simulink model "gm_UZ_EnDat"  (R2023b)
settings: Solver=FixedStepDiscrete  StartTime=0  StopTime=0.002  RelTol=1e-3
model workspace (MAT data in the model file):
  Select = 0
libraries: hdlsllib x314, hdlmdlgenlib x10, simulink x7, simulink_extras x3
(part 1 of 7)
settings Model: SimulationMode=accelerator  PacingRate=1000  Creator=ELSYS_PC  LastModifiedBy=ELSYS_PC
settings SolverCC: AlgebraicLoopSolver=TrustRegion
settings DataIOCC: LimitDataPoints=on  SaveOutput=off  SaveTime=off
settings OptimizationCC: BlockReduction=off  ConditionallyExecuteInputs=off  DefaultParameterBehavior=Inlined  InheritOutputTypeSmallerThanSingle=on  LifeSpan=inf
settings DebuggingCC: AlgebraicLoopMsg=error  InheritedTsInSrcMsg=none  SingleTaskRateTransMsg=error  UnconnectedInputMsg=warning  UnconnectedOutputMsg=warning  UnconnectedLineMsg=warning  AllowSymbolicDim=off  StrictBusMsg=ErrorOnBusTreatedAsVector  SFUnexpectedBacktrackingDiag=warning  SFNoUnconditionalDefaultTransitionDiag=warning  SFExecutionAtInitializationDiag=none  ArithmeticOperatorsInVariantConditions=warning
settings HardwareCC: ProdBitPerPointer=32  ProdBitPerSizeT=32  ProdBitPerPtrDiffT=32  ProdLargestAtomicFloat=None  ProdIntDivRoundTo=Undefined  ProdEndianess=Unspecified  ProdWordSize=32  ProdHWDeviceType=ASIC/FPGA->ASIC/FPGA  TargetBitPerPointer=64  TargetBitPerSizeT=64  TargetBitPerPtrDiffT=64  TargetLongLongMode=on  TargetIntDivRoundTo=Zero  TargetEndianess=LittleEndian  TargetWordSize=64  TargetHWDeviceType=Custom Processor->MATLAB Host Computer  ProdEqTarget=off
settings ModelReferenceCC: EnableRefExpFcnMdlSchedulingChecks=on
settings SFSimCC: SimUseLocalCustomCode=off  CustomCodeUndefinedFunction=UseInterfaceOnly
settings RTWCC: RTWUseLocalCustomCode=off
settings CodeAppCC: StateflowObjectComments=on
settings GRTTargetCC: TargetLangStandard=C89/C90 (ANSI)  RTWCAPISignals=on  RTWCAPIParams=on
settings ConfigComp: CovScope=ReferencedModels  CovMetricSettings=dw  CovSaveCumulativeToWorkspaceVar=on  CovSaveSingleToWorkspaceVar=on  CovExternalEMLEnable=off  CovSFcnEnable=off  DVTestSuiteOptimization=Auto  DVDetectOutOfBounds=on  DVModelReferenceHarness=on  DVHarnessSource=Signal Editor  DVRebuildModelRepresentation=IfChangeIsDetected

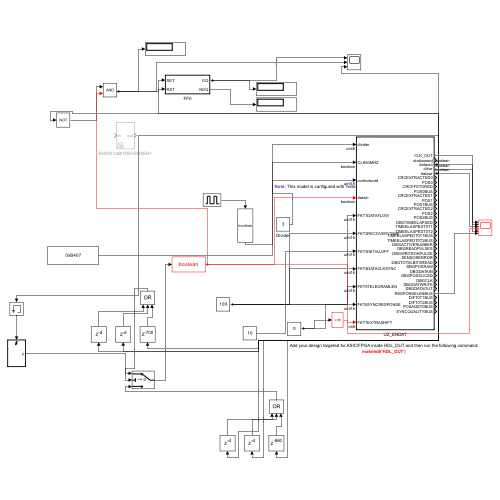
[thumbnail: Simulink's stored preview of the top-level diagram]
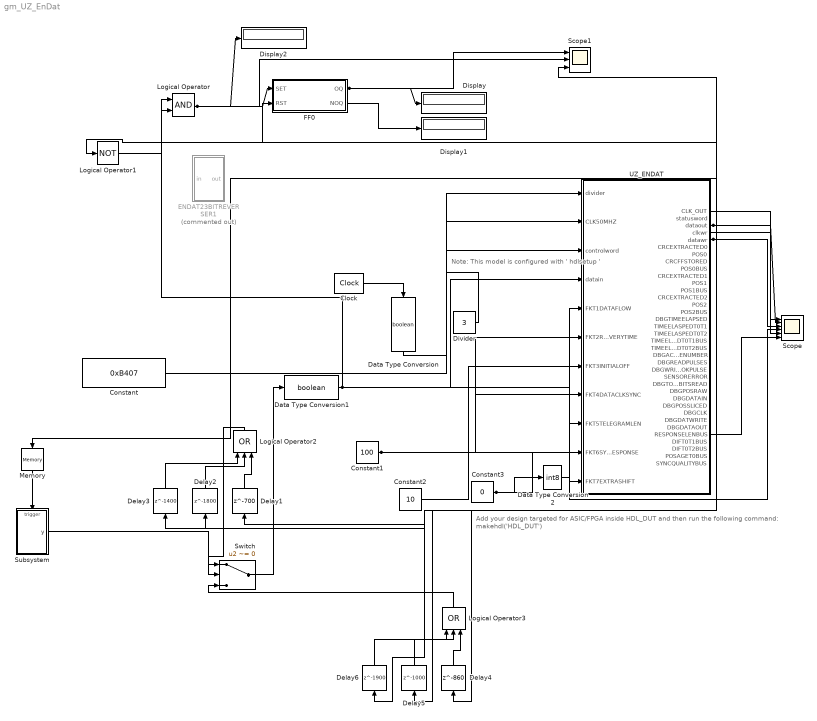
== system gm_UZ_EnDat ==
  note: Add your design targeted for ASIC/FPGA inside HDL_DUT and then run the following command:
      | makehdl('HDL_DUT')
  note: Note: This model is configured with ' hdlsetup '
  Clock : simulink_extras/Flip Flops/Clock  period=2E-8
  Constant : Constant  Value=0xB407  OutDataTypeStr=uint16  SampleTime=-1
  Constant1 : Constant  Value=100  OutDataTypeStr=uint16  SampleTime=-1
  Constant2 : Constant  Value=10  OutDataTypeStr=uint16  SampleTime=-1
  Constant3 : Constant  Value=0  OutDataTypeStr=uint16  SampleTime=-1
  Data Type Conversion : DataTypeConversion  OutDataTypeStr=boolean  SaturateOnIntegerOverflow=off  RndMeth=Floor
  Data Type Conversion1 : DataTypeConversion  OutDataTypeStr=boolean  SaturateOnIntegerOverflow=off  RndMeth=Floor
  Data Type Conversion2 : DataTypeConversion  OutDataTypeStr=int8  SaturateOnIntegerOverflow=off  RndMeth=Floor
  Delay1 : Delay  DelayLength=700
  Delay2 : Delay  DelayLength=1800
  Delay3 : Delay  DelayLength=1400
  Delay4 : Delay  DelayLength=860
  Delay5 : Delay  DelayLength=1000
  Delay6 : Delay  DelayLength=1900
  Display : Display
  Display1 : Display
  Display2 : Display
  Divider : Constant  Value=3  OutMin=0  OutMax=7  OutDataTypeStr=uint8  SampleTime=-1
  ENDAT23BITREVERSER1 : Subsystem  Commented=on
  FF0 : Subsystem  TreatAsAtomicUnit=on
      settings: LibrarySourceBlock=|
      | hdlsllib/Ports &
      | Subsystems/Triggered
      | Subsystem
  Logical Operator : Logic  AllPortsSameDT=off  OutDataTypeStr=boolean
  Logical Operator1 : Logic  Operator=NOT  AllPortsSameDT=off  OutDataTypeStr=boolean
  Logical Operator2 : Logic  Operator=OR  Inputs=3  AllPortsSameDT=off  OutDataTypeStr=boolean
  Logical Operator3 : Logic  Operator=OR  Inputs=3  AllPortsSameDT=off  OutDataTypeStr=boolean
  Memory : Memory  InheritSampleTime=on
  Scope : Scope  NumInputPorts=6
  Scope1 : Scope  NumInputPorts=3
  Subsystem : Subsystem
  Switch : Switch  Criteria=u2 ~= 0  SaturateOnIntegerOverflow=off  InputSameDT=off
  UZ_ENDAT : Subsystem  TreatAsAtomicUnit=on
  wires:
  UZ_ENDAT/32(RESPONSELENBUS) -> Scope/6
  Data Type Conversion2/1 -> UZ_ENDAT/11(FKT7EXTRASHIFT)
  Constant3/1 -> Data Type Conversion2/1, UZ_ENDAT/10(FKT6SYNCRESPONSE)
  UZ_ENDAT/4(clkwr) -> Scope/5
  Memory/1 -> Subsystem/Trigger
  Subsystem/1(y) -> Switch/2
  UZ_ENDAT/3(dataout) -> Scope/2, Delay5/1, Delay1/1, Delay2/1, Delay3/1, Delay6/1, Delay4/1
  Delay4/1 -> Logical Operator3/3
  Logical Operator3/1 -> Switch/3
  Delay5/1 -> Logical Operator3/2
  Delay6/1 -> Logical Operator3/1
  Switch/1 -> Data Type Conversion1/1
  Logical Operator2/1 -> Switch/1
  Delay3/1 -> Logical Operator2/1
  Delay2/1 -> Logical Operator2/2
  Logical Operator1/1 -> Logical Operator/1
  FF0/2(NOQ) -> Display1/1
  Logical Operator/1 -> Display2/1, FF0/1(SET), Scope1/2
  FF0/1(OQ) -> Display/1, Scope1/1
  Constant2/1 -> UZ_ENDAT/7(FKT3INITIALOFF)
  Constant1/1 -> UZ_ENDAT/9(FKT5TELEGRAMLEN), UZ_ENDAT/8(FKT4DATACLKSYNC), UZ_ENDAT/6(FKT2RECOVERYTIME), UZ_ENDAT/5(FKT1DATAFLOW)
  UZ_ENDAT/5(datawr) -> Scope/3, Logical Operator1/1, FF0/2(RST), Scope1/3, Memory/1
  UZ_ENDAT/1(CLK_OUT) -> Scope/1
  Delay1/1 -> Logical Operator2/3
  Data Type Conversion1/1 -> UZ_ENDAT/4(datain), Scope/4, Logical Operator/2
  Clock/1 -> Data Type Conversion/1
  Divider/1 -> UZ_ENDAT/1(divider)
  Data Type Conversion/1 -> UZ_ENDAT/2(CLK50MHZ)
  Constant/1 -> UZ_ENDAT/3(controlword)

== system gm_UZ_EnDat/ENDAT23BITREVERSER1 ==
  in : Inport
  16BITREVERSER : Subsystem
  16BITREVERSER1 : Subsystem
  Bit Concat : hdlsllib/Logic and Bit Operations/Bit Concat  numInputs=2
  Bit Shift : hdlsllib/Logic and Bit Operations/Bit Shift  mode=Shift Right Logical  N=8
  Bit Slice : hdlsllib/Logic and Bit Operations/Bit Slice  lidx=15  ridx=0
  Bit Slice1 : hdlsllib/Logic and Bit Operations/Bit Slice  lidx=22  ridx=16
  out : Outport
  wires:
  16BITREVERSER1/1(out) -> Bit Concat/2
  16BITREVERSER/1(out) -> Bit Concat/1
  Bit Slice1/1 -> 16BITREVERSER1/1(in)
  Bit Slice/1 -> 16BITREVERSER/1(in)
  in/1 -> Bit Slice/1, Bit Slice1/1
  Bit Shift/1 -> out/1
  Bit Concat/1 -> Bit Shift/1

== system gm_UZ_EnDat/FF0 ==
  SET : Inport
  RST : Inport  Port=2
  S-R Flip-Flop : simulink_extras/Flip Flops/S-R Flip-Flop  initial_condition=0
  OQ : Outport
  NOQ : Outport  Port=2
  wires:
  S-R Flip-Flop/2 -> NOQ/1
  S-R Flip-Flop/1 -> OQ/1
  RST/1 -> S-R Flip-Flop/2
  SET/1 -> S-R Flip-Flop/1

== system gm_UZ_EnDat/Subsystem ==
  Trigger : TriggerPort  VariantControl=(inherit)  PortDimensions=1
  Counter Limited : hdlsllib/Sources/Counter Limited  uplimit=1  tsamp=-1
  y : Outport
  wires:
  Counter Limited/1 -> y/1

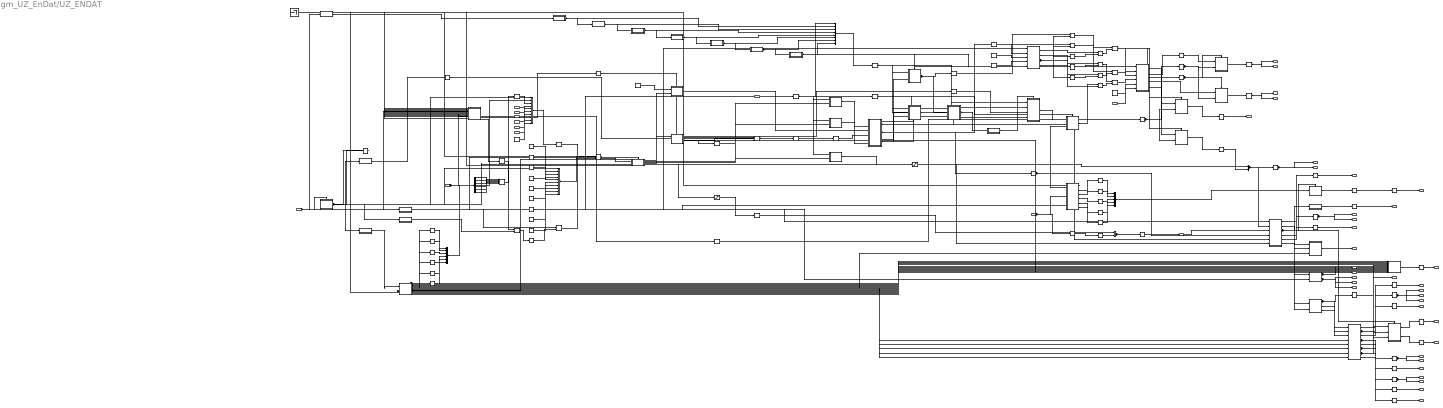
== system gm_UZ_EnDat/UZ_ENDAT ==
  note: 0=12.5;1=6,25;2=3,125;3=1,5625
  divider : Inport  OutDataTypeStr=uint8  PortDimensions=1  SampleTime=1e-08
  CLK50MHZ : Inport  Port=2  OutDataTypeStr=boolean  PortDimensions=1  SampleTime=1e-08
  controlword : Inport  Port=3  OutDataTypeStr=uint16  PortDimensions=1  SampleTime=1e-08
  datain : Inport  Port=4  OutDataTypeStr=boolean  PortDimensions=1  SampleTime=1e-08
  FKT1DATAFLOW : Inport  Port=5  OutDataTypeStr=uint16  PortDimensions=1  SampleTime=1e-08
  FKT2RECOVERYTIME : Inport  Port=6  OutDataTypeStr=uint16  PortDimensions=1  SampleTime=1e-08
  FKT3INITIALOFF : Inport  Port=7  OutDataTypeStr=uint16  PortDimensions=1  SampleTime=1e-08
  FKT4DATACLKSYNC : Inport  Port=8  OutDataTypeStr=uint16  PortDimensions=1  SampleTime=1e-08
  FKT5TELEGRAMLEN : Inport  Port=9  OutDataTypeStr=uint16  PortDimensions=1  SampleTime=1e-08
  FKT6SYNCRESPONSE : Inport  Port=10  OutDataTypeStr=uint16  PortDimensions=1  SampleTime=1e-08
  FKT7EXTRASHIFT : Inport  Port=11  OutDataTypeStr=int8  PortDimensions=1  SampleTime=1e-08
  16bitgather : Subsystem
  2CLKDELAY : simulink/Discrete/Tapped Delay  vinit=0  samptime=-1  NumDelays=double(127)  DelayOrder=Newest  includeCurrent=on
  3timestorage : Subsystem
  8BIT_SPLITTER : Subsystem
  8BIT_SPLITTER_term8 : Terminator
  CLKCNTER_ACT : Subsystem
  CLKCNTER_NOSTOP : Subsystem
  CLKDIV1 : Subsystem
  CLKDIV3 : Subsystem
  CLKDIV4 : Subsystem
  CLKDIV5 : Subsystem
  CLKDIV6 : Subsystem
  CLKDIV7 : Subsystem
  CLKDIV8 : Subsystem
  CLKDIV9 : Subsystem
  CONTROLWORDRAW : Subsystem
  CONTROLWORDRAW_term{0..11,14} (13 alike) : Terminator
  CONTROLWORDSTORED : Subsystem
  CONTROLWORDSTORED_term13 : Terminator
  CRC_Check : Subsystem
  CRC_Check_term0 : Terminator
  Compare To Constant : Subsystem  mask(Compare To Constant){relop===, const=double(1), OutDataTypeStr=boolean, ZeroCross=on}
      mask prompts: relop "Simulink:masks:Operator_MP"; const "Simulink:masks:ConstantValue_MP"; OutDataTypeStr "Simulink:masks:OutputDataType_MP"; ZeroCross "Simulink:masks:EnableZerocrossingDetection_MP"
      mask help: Simulink:masks:CompareToConstant_MD
      mask init:
      | OutDataTypeStr = 'boolean';
      | ZeroCross = 'on';
      | blkName = 'UZ_EnDat/UZ_ENDAT/Compare\nTo Constant';
      | const = double(1);
      | const_str = '1';
      | const_val = double(1);
      | relop = '==';
      | setValue = 'boolean';
      | str = '== 1';
      mask TypeOptions relop: == | ~= | < | <= | >= | >
      mask TypeOptions OutDataTypeStr: Simulink:masks:uint8 | Simulink:masks:boolean
      mask Callback ZeroCross: sl('zeroCrossEnable', gcbh);
      mask Display: disp(str)
  Compare To Constant1 : Subsystem  mask(Compare To Constant){relop===, const=double(1), OutDataTypeStr=boolean, ZeroCross=on}
      mask prompts: relop "Simulink:masks:Operator_MP"; const "Simulink:masks:ConstantValue_MP"; OutDataTypeStr "Simulink:masks:OutputDataType_MP"; ZeroCross "Simulink:masks:EnableZerocrossingDetection_MP"
      mask help: Simulink:masks:CompareToConstant_MD
      mask init:
      | OutDataTypeStr = 'boolean';
      | ZeroCross = 'on';
      | blkName = 'UZ_EnDat/UZ_ENDAT/Compare\nTo Constant1';
      | const = double(1);
      | const_str = '1';
      | const_val = double(1);
      | relop = '==';
      | setValue = 'boolean';
      | str = '== 1';
      mask TypeOptions relop: == | ~= | < | <= | >= | >
      mask TypeOptions OutDataTypeStr: Simulink:masks:uint8 | Simulink:masks:boolean
      mask Callback ZeroCross: sl('zeroCrossEnable', gcbh);
      mask Display: disp(str)
  Compare To Constant2 : Subsystem  mask(Compare To Constant){relop===, const=double(0), OutDataTypeStr=boolean, ZeroCross=on}
      mask prompts: relop "Simulink:masks:Operator_MP"; const "Simulink:masks:ConstantValue_MP"; OutDataTypeStr "Simulink:masks:OutputDataType_MP"; ZeroCross "Simulink:masks:EnableZerocrossingDetection_MP"
      mask help: Simulink:masks:CompareToConstant_MD
      mask init:
      | OutDataTypeStr = 'boolean';
      | ZeroCross = 'on';
      | blkName = 'UZ_EnDat/UZ_ENDAT/Compare\nTo Constant2';
      | const = double(0);
      | const_str = '0';
      | const_val = double(0);
      | relop = '==';
      | setValue = 'boolean';
      | str = '== 0';
      mask TypeOptions relop: == | ~= | < | <= | >= | >
      mask TypeOptions OutDataTypeStr: Simulink:masks:uint8 | Simulink:masks:boolean
      mask Callback ZeroCross: sl('zeroCrossEnable', gcbh);
      mask Display: disp(str)
  Compare To Constant3 : Subsystem  mask(Compare To Constant){relop=>=, const=double(3), OutDataTypeStr=boolean, ZeroCross=on}
      mask prompts: relop "Simulink:masks:Operator_MP"; const "Simulink:masks:ConstantValue_MP"; OutDataTypeStr "Simulink:masks:OutputDataType_MP"; ZeroCross "Simulink:masks:EnableZerocrossingDetection_MP"
      mask help: Simulink:masks:CompareToConstant_MD
      mask init:
      | OutDataTypeStr = 'boolean';
      | ZeroCross = 'on';
      | blkName = 'UZ_EnDat/UZ_ENDAT/Compare\nTo Constant3';
      | const = double(3);
      | const_str = '3';
      | const_val = double(3);
      | relop = '>=';
      | setValue = 'boolean';
      | str = '>= 3';
      mask TypeOptions relop: == | ~= | < | <= | >= | >
      mask TypeOptions OutDataTypeStr: Simulink:masks:uint8 | Simulink:masks:boolean
      mask Callback ZeroCross: sl('zeroCrossEnable', gcbh);
      mask Display: disp(str)
  Constant3 : Constant  OutDataTypeStr=boolean  SampleTime=1e-08
  Constant6 : Constant  Value=51  OutDataTypeStr=uint16  SampleTime=1e-08
  ControlWordRAM : Constant  Value=0  VectorParams1D=off  OutDataTypeStr=uint8  SampleTime=1e-08
  DATA2CLOCKSYNCER : Subsystem
  DATAFLOWCHGER : Subsystem
  DIFFBUILDER : Subsystem
  Data Type Conversion : DataTypeConversion  OutDataTypeStr=fixdt(0, 4, 0)  RndMeth=Nearest  SampleTime=1e-08
  Data Type Conversion1 : DataTypeConversion  OutDataTypeStr=uint8  SampleTime=1e-08  SaturateOnIntegerOverflow=off  RndMeth=Floor
  Data Type Conversion{2..12} (11 alike) : DataTypeConversion  OutDataTypeStr=fixdt(0, 1, 0)  SampleTime=1e-08  SaturateOnIntegerOverflow=off  RndMeth=Floor
  Delay1 : simulink/Discrete/Tapped Delay  vinit=0  samptime=-1  NumDelays=double(127)  DelayOrder=Newest  includeCurrent=on
  Delay4 : hdlmdlgenlib/Buffer
  Detect Change : Subsystem  mask(Detect Change){vinit=double(0), InputProcessing=Elements as channels (sample based), OutDataTypeStr=boolean}
      mask prompts: vinit "Simulink:masks:InitialCondition_MP"; InputProcessing "Simulink:masks:InputProcessing_MP"; OutDataTypeStr "Simulink:masks:OutputDataType_MP"
      mask help: Simulink:masks:DetectChange_MD
      mask init:
      | InputProcessing = 'Elements as channels (sample based)';
      | OutDataTypeStr = 'boolean';
      | vinit = double(0);
      mask TypeOptions InputProcessing: Simulink:masks:ColumnsAsChannelsFrameBased | Simulink:masks:ElementsAsChannelsSampleBased
      mask TypeOptions OutDataTypeStr: Simulink:masks:uint8 | Simulink:masks:boolean
      mask Display: fprintf('U ~= U/z')
  Dual Port RAM System : hdlsllib/HDL RAMs/Dual Port RAM System  RAMType=Dual port  AsyncRead=off  WriteOutputValue=New data  RAMInitialValue=0  allowBusInputs=off  WritesHaveOutput=on  NumReads=0  NumWrites=1  SimulateUsing=Code generation
  Dual Port RAM System_term0 : Terminator
  EndatControlRAM : Constant  VectorParams1D=off  OutDataTypeStr=uint8  SampleTime=1e-08
  FKT1 : Constant  Value=2  VectorParams1D=off  OutDataTypeStr=uint8  SampleTime=1e-08
  FKT2 : Constant  Value=3  VectorParams1D=off  OutDataTypeStr=uint8  SampleTime=1e-08
  FKT4 : Constant  Value=5  VectorParams1D=off  OutDataTypeStr=uint8  SampleTime=1e-08
  FKT5 : Constant  Value=6  VectorParams1D=off  OutDataTypeStr=uint8  SampleTime=1e-08
  FKT6 : Constant  Value=7  VectorParams1D=off  OutDataTypeStr=uint8  SampleTime=1e-08
  FKT7 : Constant  Value=8  VectorParams1D=off  OutDataTypeStr=uint8  SampleTime=1e-08
  INITIALOFF : Subsystem
  Logical Operator{,1,9,13..14,16,18,20} (8 alike) : Logic  AllPortsSameDT=off  OutDataTypeStr=boolean  SampleTime=1e-08
  Logical Operator{2..4,6,10,17,19,21,27} (9 alike) : Logic  Operator=NOT  Inputs=1  AllPortsSameDT=off  OutDataTypeStr=boolean  SampleTime=1e-08
  Logical Operator15 : Logic  Operator=OR  AllPortsSameDT=off  OutDataTypeStr=boolean  SampleTime=1e-08
  Logical Operator22 : Logic  Operator=OR  AllPortsSameDT=off  OutDataTypeStr=boolean  SampleTime=1e-08
  Logical Operator23 : Logic  Operator=OR  AllPortsSameDT=off  OutDataTypeStr=boolean  SampleTime=1e-08
  Logical Operator8 : Logic  Inputs=3  AllPortsSameDT=off  OutDataTypeStr=boolean  SampleTime=1e-08
  ManualSerialize : Subsystem
  Multiport Switch : MultiPortSwitch  DataPortOrder=Zero-based contiguous  Inputs=7  DiagnosticForDefault=None  zeroidx=on  SampleTime=1e-08  SaturateOnIntegerOverflow=off  InputSameDT=off
  OUTPUTCONTROLCONTINIOUS : Subsystem
  RAM_SELECTOR : MultiPortSwitch  DataPortOrder=Zero-based contiguous  Inputs=8  DataPortForDefault=Additional data port  DiagnosticForDefault=None  zeroidx=on  OutDataTypeStr=uint8  SampleTime=1e-08  SaturateOnIntegerOverflow=off  InputSameDT=off
  RAM_SELECTOR1 : MultiPortSwitch  DataPortOrder=Zero-based contiguous  Inputs=8  DataPortForDefault=Additional data port  DiagnosticForDefault=None  zeroidx=on  OutDataTypeStr=uint16  SampleTime=1e-08  SaturateOnIntegerOverflow=off  InputSameDT=off
  RECOVERYTIMESELECTOR : Subsystem
  RESPONSESLICER3X : Subsystem
  SetZeroBool : Subsystem
  SetZeroBool1 : Subsystem
  SetZeroBool2 : Subsystem
  SetZeroBool3 : Subsystem
  SetZeroBool4 : Subsystem
  SetZeroBool5 : Subsystem
  Signal Specification : SignalSpecification  OutDataTypeStr=uint16  Dimensions=1
  Storage16 : Subsystem
  Subsystem : Subsystem
  Subsystem1 : Subsystem
  Subsystem2 : Subsystem
  Subsystem6 : Subsystem
  TmpGroundAtRAM_SELECTOR1Inport10 : Constant  Value=0  VectorParams1D=off  OutDataTypeStr=uint16  SampleTime=1e-08
  TmpGroundAtRAM_SELECTORInport10 : Constant  Value=0  VectorParams1D=off  OutDataTypeStr=uint8  SampleTime=1e-08
  ageprovider : Subsystem
  concat : hdlsllib/Logic and Bit Operations/Bit Concat  numInputs=6
  concatenate : Concatenate  NumInputs=5
  concatenate1 : Concatenate  NumInputs=6
  multiportswitch : MultiPortSwitch  DataPortOrder=Zero-based contiguous  Inputs=1  DiagnosticForDefault=None  zeroidx=on  SampleTime=1e-08  SaturateOnIntegerOverflow=off  InputSameDT=off
  multiportswitch1 : MultiPortSwitch  DataPortOrder=Zero-based contiguous  Inputs=1  DiagnosticForDefault=None  zeroidx=on  SampleTime=1e-08  SaturateOnIntegerOverflow=off  InputSameDT=off
  ramselektor : Subsystem
  rd_{0,4..5,10..11,13..15,17..18} (10 alike) : Delay  DelayLength=double(1)  InitialCondition=0  SampleTime=1e-08
  rd_1 : Delay  DelayLength=double(10)  InitialCondition=0  SampleTime=1e-08
  rd_{2..3,6..9,12,16,19..25,27..31,33..35} (23 alike) : Delay  DelayLength=double(2)  InitialCondition=0  SampleTime=1e-08
  rd_26 : Delay  DelayLength=double(4)  InitialCondition=0  SampleTime=1e-08
  rd_32 : Delay  DelayLength=double(3)  InitialCondition=0  SampleTime=1e-08
  saturate : Saturate  UpperLimit=double(127)  LowerLimit=double(0)  SampleTime=1e-08  OutDataTypeStr=uint16
  saturate1 : Saturate  UpperLimit=double(127)  LowerLimit=double(0)  SampleTime=1e-08  OutDataTypeStr=uint16
  signalquality : Subsystem
  t : Constant  Value=double(0)  OutDataTypeStr=boolean  SampleTime=1e-08
  t1 : Constant  Value=fi(0,0,8,0)  OutDataTypeStr=uint8  SampleTime=1e-08
  t2 : Constant  Value=fi(0,0,16,0)  OutDataTypeStr=uint16  SampleTime=1e-08
  t3 : Demux  Outputs=6
  timingprovider : Subsystem
  CLK_OUT : Outport  SampleTime=1e-08  VectorParamsAs1DForOutWhenUnconnected=off
  statusword : Outport  Port=2  OutDataTypeStr=uint16  SampleTime=1e-08  VectorParamsAs1DForOutWhenUnconnected=off
  dataout : Outport  Port=3  OutDataTypeStr=boolean  SampleTime=1e-08  VectorParamsAs1DForOutWhenUnconnected=off
  clkwr : Outport  Port=4  OutDataTypeStr=boolean  SampleTime=1e-08  VectorParamsAs1DForOutWhenUnconnected=off
  datawr : Outport  Port=5  OutDataTypeStr=boolean  SampleTime=1e-08  VectorParamsAs1DForOutWhenUnconnected=off
  CRCEXTRACTED0 : Outport  Port=6  OutDataTypeStr=uint8  SampleTime=1e-08  VectorParamsAs1DForOutWhenUnconnected=off
  POS0 : Outport  Port=7  OutDataTypeStr=uint32  SampleTime=1e-08  VectorParamsAs1DForOutWhenUnconnected=off
  CRCFFSTORED : Outport  Port=8  OutDataTypeStr=uint8  SampleTime=1e-08  VectorParamsAs1DForOutWhenUnconnected=off
  POS0BUS : Outport  Port=9  OutDataTypeStr=uint32  SampleTime=1e-08  VectorParamsAs1DForOutWhenUnconnected=off
  CRCEXTRACTED1 : Outport  Port=10  OutDataTypeStr=uint8  SampleTime=1e-08  VectorParamsAs1DForOutWhenUnconnected=off
  POS1 : Outport  Port=11  OutDataTypeStr=uint32  SampleTime=1e-08  VectorParamsAs1DForOutWhenUnconnected=off
  POS1BUS : Outport  Port=12  OutDataTypeStr=uint32  SampleTime=1e-08  VectorParamsAs1DForOutWhenUnconnected=off
  CRCEXTRACTED2 : Outport  Port=13  OutDataTypeStr=uint8  SampleTime=1e-08  VectorParamsAs1DForOutWhenUnconnected=off
  POS2 : Outport  Port=14  OutDataTypeStr=uint32  SampleTime=1e-08  VectorParamsAs1DForOutWhenUnconnected=off
  POS2BUS : Outport  Port=15  OutDataTypeStr=uint32  SampleTime=1e-08  VectorParamsAs1DForOutWhenUnconnected=off
  DBGTIMEELAPSED : Outport  Port=16  SampleTime=1e-08  VectorParamsAs1DForOutWhenUnconnected=off
  TIMEELASPEDT0T1 : Outport  Port=17  SampleTime=1e-08  VectorParamsAs1DForOutWhenUnconnected=off
  TIMEELASPEDT0T2 : Outport  Port=18  SampleTime=1e-08  VectorParamsAs1DForOutWhenUnconnected=off
  TIMEELASPEDT0T1BUS : Outport  Port=19  SampleTime=1e-08  VectorParamsAs1DForOutWhenUnconnected=off
  TIMEELASPEDT0T2BUS : Outport  Port=20  SampleTime=1e-08  VectorParamsAs1DForOutWhenUnconnected=off
  DBGACTIVENUMBER : Outport  Port=21  OutDataTypeStr=uint8  SampleTime=1e-08  VectorParamsAs1DForOutWhenUnconnected=off
  DBGREADPULSES : Outport  Port=22  OutDataTypeStr=boolean  SampleTime=1e-08  VectorParamsAs1DForOutWhenUnconnected=off
  DBGWRITEOKPULSE : Outport  Port=23  OutDataTypeStr=boolean  SampleTime=1e-08  VectorParamsAs1DForOutWhenUnconnected=off
  SENSORERROR : Outport  Port=24  OutDataTypeStr=boolean  SampleTime=1e-08  VectorParamsAs1DForOutWhenUnconnected=off
  DBGTOTALBITSREAD : Outport  Port=25  SampleTime=1e-08  VectorParamsAs1DForOutWhenUnconnected=off
  DBGPOSRAW : Outport  Port=26  OutDataTypeStr=uint64  SampleTime=1e-08  VectorParamsAs1DForOutWhenUnconnected=off
  DBGDATAIN : Outport  Port=27  OutDataTypeStr=boolean  SampleTime=1e-08  VectorParamsAs1DForOutWhenUnconnected=off
  DBGPOSSLICED : Outport  Port=28  OutDataTypeStr=uint32  SampleTime=1e-08  VectorParamsAs1DForOutWhenUnconnected=off
  DBGCLK : Outport  Port=29  SampleTime=1e-08  VectorParamsAs1DForOutWhenUnconnected=off
  DBGDATWRITE : Outport  Port=30  SampleTime=1e-08  VectorParamsAs1DForOutWhenUnconnected=off
  DBGDATAOUT : Outport  Port=31  OutDataTypeStr=boolean  SampleTime=1e-08  VectorParamsAs1DForOutWhenUnconnected=off
  RESPONSELENBUS : Outport  Port=32  SampleTime=1e-08  VectorParamsAs1DForOutWhenUnconnected=off
  DIFT0T1BUS : Outport  Port=33  OutDataTypeStr=int32  SampleTime=1e-08  VectorParamsAs1DForOutWhenUnconnected=off
  DIFT0T2BUS : Outport  Port=34  OutDataTypeStr=int32  SampleTime=1e-08  VectorParamsAs1DForOutWhenUnconnected=off
  POSAGET0BUS : Outport  Port=35  SampleTime=1e-08  VectorParamsAs1DForOutWhenUnconnected=off
  SYNCQUALITYBUS : Outport  Port=36  SampleTime=1e-08  VectorParamsAs1DForOutWhenUnconnected=off
  wires:
  divider/1 -> Data Type Conversion/1
  controlword/1 -> CONTROLWORDRAW/2(DATA), RAM_SELECTOR1/2
  datain/1 -> Delay1/1, CRC_Check/2(data)
  FKT3INITIALOFF/1 -> INITIALOFF/6(FACTOR)
  16bitgather/1(statusword) -> rd_12/1
  3timestorage/2(t-1) -> RESPONSESLICER3X/2(DATA1)
  3timestorage/3(t-2) -> RESPONSESLICER3X/3(DATA2)
  8BIT_SPLITTER/2(DATAOUT1) -> Storage16/1(Data)
  8BIT_SPLITTER/3(DATAOUT2) -> DATAFLOWCHGER/2(FACTOR)
  8BIT_SPLITTER/4(DATAOUT3) -> RECOVERYTIMESELECTOR/2(FAKTOR)
  8BIT_SPLITTER/5(DATAOUT4) -> DATA2CLOCKSYNCER/2(FAKTOR)
  8BIT_SPLITTER/6(DATAOUT5) -> Subsystem6/2(FACTOR)
  8BIT_SPLITTER/7(DATAOUT6) -> saturate1/1
  8BIT_SPLITTER/8(DATAOUT7) -> ManualSerialize/6(FKT7EXTRASHIFTER)
  CLKDIV1/1(CLK/2) -> CLKDIV3/1(CLK1)
  CLKDIV3/1(CLK/2) -> Multiport Switch/2, CLKDIV4/1(CLK1)
  CLKDIV4/1(CLK/2) -> Multiport Switch/3, CLKDIV5/1(CLK1)
  CLKDIV5/1(CLK/2) -> Multiport Switch/4, CLKDIV6/1(CLK1)
  CLKDIV6/1(CLK/2) -> Multiport Switch/5, CLKDIV7/1(CLK1)
  CLKDIV7/1(CLK/2) -> Multiport Switch/6, CLKDIV8/1(CLK1)
  CLKDIV8/1(CLK/2) -> Multiport Switch/7, CLKDIV9/1(CLK1)
  CLKDIV9/1(CLK/2) -> Multiport Switch/8, Subsystem/5(VERYSLOWCLK), INITIALOFF/1(CLKAUX)
  CONTROLWORDRAW/13(DATAOUT12) -> Logical Operator27/1
  CONTROLWORDRAW/14(DATAOUT13) -> rd_4/1
  CONTROLWORDRAW/16(DATAOUT15) -> Logical Operator3/1
  CONTROLWORDSTORED/1(DATAOUT0) -> 16bitgather/1(in1), Data Type Conversion4/1
  CONTROLWORDSTORED/2(DATAOUT1) -> 16bitgather/2(DATAOUT1), Data Type Conversion5/1
  CONTROLWORDSTORED/3(DATAOUT2) -> 16bitgather/3(DATAOUT3), Data Type Conversion6/1
  CONTROLWORDSTORED/4(DATAOUT3) -> 16bitgather/4(DATAOUT4), Data Type Conversion7/1
  CONTROLWORDSTORED/5(DATAOUT4) -> 16bitgather/5(DATAOUT5), Data Type Conversion8/1
  CONTROLWORDSTORED/7(DATAOUT6) -> 16bitgather/7(DATAOUT7), ageprovider/3(altmode)
  CONTROLWORDSTORED/8(DATAOUT7) -> 16bitgather/8(DATAOUT8), RESPONSESLICER3X/4(19BIT)
  CONTROLWORDSTORED/9(DATAOUT8) -> RESPONSESLICER3X/5(21BIT), 16bitgather/9(DATAOUT9)
  CONTROLWORDSTORED/10(DATAOUT9) -> RESPONSESLICER3X/6(23BIT), 16bitgather/10(DATAOUT10)
  CONTROLWORDSTORED/11(DATAOUT10) -> 16bitgather/11(In11), RESPONSESLICER3X/7(25BIT)
  CONTROLWORDSTORED/12(DATAOUT11) -> RESPONSESLICER3X/8(27BIT), 16bitgather/12(DATAOUT11)
  CONTROLWORDSTORED/13(DATAOUT12) -> 16bitgather/13(DATAOUT12)
  CONTROLWORDSTORED/15(DATAOUT14) -> 16bitgather/15(DATAOUT14)
  CONTROLWORDSTORED/16(DATAOUT15) -> 16bitgather/16(DATAOUT15)
  CRC_Check/2(CRC1) -> Data Type Conversion2/1
  CRC_Check/3(CRC2) -> Data Type Conversion3/1
  CRC_Check/4(CRC3) -> Data Type Conversion10/1
  CRC_Check/5(CRC4) -> Data Type Conversion11/1
  CRC_Check/6(CRC5) -> Data Type Conversion12/1
  Compare To Constant/1(y) -> Logical Operator1/2
  Compare To Constant1/1(y) -> rd_5/1
  Compare To Constant3/1(y) -> Subsystem2/Enable
  Constant3/1 -> INITIALOFF/5(CLKWR)
  Constant6/1 -> Subsystem6/1(In1)
  ControlWordRAM/1 -> RAM_SELECTOR/2
  DATA2CLOCKSYNCER/1(Out1) -> saturate/1
  Data Type Conversion/1 -> Multiport Switch/1, DATA2CLOCKSYNCER/1(In1), DATAFLOWCHGER/1(CLKSEL), RECOVERYTIMESELECTOR/1(In1)
  Data Type Conversion10/1 -> concatenate/3
  Data Type Conversion11/1 -> concatenate/4
  Data Type Conversion12/1 -> concatenate/5
  Data Type Conversion2/1 -> concatenate/1
  Data Type Conversion3/1 -> concatenate/2
  Delay4/1 -> Logical Operator13/1
  Detect Change/1(Y) -> Logical Operator/1
  Dual Port RAM System/1 -> Dual Port RAM System_term0/1
  EndatControlRAM/1 -> RAM_SELECTOR/3
  FKT1/1 -> RAM_SELECTOR/4
  FKT2/1 -> RAM_SELECTOR/5
  FKT4/1 -> RAM_SELECTOR/6
  FKT5/1 -> RAM_SELECTOR/7
  FKT6/1 -> RAM_SELECTOR/8
  FKT7/1 -> RAM_SELECTOR/9
  INITIALOFF/1(CLK_OUT) -> SetZeroBool5/1(valin)
  INITIALOFF/2(DATAWR_OUT) -> rd_17/1
  INITIALOFF/3(DATA_OUT) -> SetZeroBool3/1(valin)
  INITIALOFF/4(CLKWR_OUT) -> SetZeroBool2/1(valin)
  Logical Operator1/1 -> Logical Operator2/1
  Logical Operator13/1 -> Logical Operator22/1
  Logical Operator14/1 -> Logical Operator15/1
  Logical Operator15/1 -> INITIALOFF/3(DATAWR)
  Logical Operator16/1 -> Logical Operator15/2
  Logical Operator17/1 -> Logical Operator16/2
  Logical Operator18/1 -> Logical Operator22/2
  Logical Operator19/1 -> Logical Operator18/2
  Logical Operator2/1 -> Logical Operator/2
  Logical Operator20/1 -> Logical Operator23/1
  Logical Operator21/1 -> Logical Operator20/2
  Logical Operator23/1 -> INITIALOFF/4(DATA)
  Logical Operator3/1 -> Logical Operator1/1
  Logical Operator4/1 -> ManualSerialize/4(recieving), CRC_Check/1(set), SetZeroBool1/2(setzero)
  Logical Operator8/1 -> Logical Operator10/1, Storage16/2(Write)
  Logical Operator9/1 -> Logical Operator23/2
  ManualSerialize/2(valueout) -> 3timestorage/1(DATA)
  ManualSerialize/3(wrok) -> Subsystem1/Enable, 3timestorage/2(wrok), signalquality/1(wrok), DIFFBUILDER/Trigger, ageprovider/1(wrok), timingprovider/1(wrok)
  ManualSerialize/6(beginrecieving) -> ageprovider/2(recieving)
  SetZeroBool1/1(valueout) -> Logical Operator9/1
  SetZeroBool5/1(valueout) -> 2CLKDELAY/1
  Storage16/2(wrok) -> 16bitgather/14(wrok), Logical Operator6/1
  Subsystem/1(CLKOUT) -> Logical Operator18/1
  Subsystem/2(DATAOUT) -> Logical Operator20/1
  Subsystem/3(BOOTUPCOMPLETE) -> Logical Operator9/2, Logical Operator21/1, Logical Operator19/1, Logical Operator17/1, Logical Operator14/2, Logical Operator13/2
  Subsystem/4(DATAINV) -> Logical Operator16/1
  Subsystem1/1(out) -> Data Type Conversion1/1
  Subsystem2/1(valin) -> SetZeroBool1/1(valin)
  TmpGroundAtRAM_SELECTORInport10/1 -> RAM_SELECTOR/10
  concatenate/1 -> Subsystem1/1(in)
  ageprovider/1(posage) -> POSAGET0BUS/1
  ramselektor/1(SEL) -> rd_0/1, RAM_SELECTOR/1, Compare To Constant/1(u), Detect Change/1(U), Compare To Constant2/1(u), Compare To Constant1/1(u), 8BIT_SPLITTER/2(SEL), RAM_SELECTOR1/1
  timingprovider/1(timeelapsed2cycl) -> TIMEELASPEDT0T2BUS/1, TIMEELASPEDT0T2/1
  timingprovider/2(timeelapsed1cycl) -> DBGTIMEELAPSED/1, TIMEELASPEDT0T1/1, TIMEELASPEDT0T1BUS/1
  2CLKDELAY/1 -> multiportswitch/2
  saturate/1 -> multiportswitch/1
  Delay1/1 -> rd_11/1
  saturate1/1 -> rd_10/1
  8BIT_SPLITTER/9(DATAOUT8) -> 8BIT_SPLITTER_term8/1
  CONTROLWORDRAW/1(DATAOUT0) -> CONTROLWORDRAW_term0/1
  CONTROLWORDRAW/2(DATAOUT1) -> CONTROLWORDRAW_term1/1
  CONTROLWORDRAW/3(DATAOUT2) -> CONTROLWORDRAW_term2/1
  CONTROLWORDRAW/4(DATAOUT3) -> CONTROLWORDRAW_term3/1
  CONTROLWORDRAW/5(DATAOUT4) -> CONTROLWORDRAW_term4/1
  CONTROLWORDRAW/6(DATAOUT5) -> CONTROLWORDRAW_term5/1
  CONTROLWORDRAW/7(DATAOUT6) -> CONTROLWORDRAW_term6/1
  CONTROLWORDRAW/8(DATAOUT7) -> CONTROLWORDRAW_term7/1
  CONTROLWORDRAW/9(DATAOUT8) -> CONTROLWORDRAW_term8/1
  CONTROLWORDRAW/10(DATAOUT9) -> CONTROLWORDRAW_term9/1
  CONTROLWORDRAW/11(DATAOUT10) -> CONTROLWORDRAW_term10/1
  CONTROLWORDRAW/12(DATAOUT11) -> CONTROLWORDRAW_term11/1
  CONTROLWORDRAW/15(DATAOUT14) -> CONTROLWORDRAW_term14/1
  CONTROLWORDSTORED/14(DATAOUT13) -> CONTROLWORDSTORED_term13/1
  CRC_Check/1(crc) -> CRC_Check_term0/1
  t/1 -> Subsystem/2(RESET)
  t1/1 -> Subsystem/3(CLKS2DATAFLOWCHG)
  t2/1 -> Subsystem/4(CLK2ENDOFTRANSMISSION)
  Logical Operator10/1 -> rd_6/1
  Storage16/1(out) -> rd_7/1
  SetZeroBool2/1(valueout) -> rd_16/1
  RESPONSESLICER3X/1(CRC) -> rd_19/1
  Data Type Conversion1/1 -> rd_21/1
  RESPONSESLICER3X/3(CRC1) -> rd_22/1
  RESPONSESLICER3X/5(CRC2) -> rd_24/1
  RESPONSESLICER3X/8(DBGACTIVENUMBER) -> rd_26/1
  ManualSerialize/1(dbg) -> rd_27/1
  ManualSerialize/5(dbg1) -> rd_28/1
  RESPONSESLICER3X/7(sensorerror) -> rd_29/1, 16bitgather/6(DATAOUT6)
  3timestorage/1(t0) -> rd_31/1, RESPONSESLICER3X/1(DATA)
  multiportswitch1/1 -> rd_32/1, ManualSerialize/3(DATA)
  DIFFBUILDER/1(DIFT1T0) -> rd_33/1
  DIFFBUILDER/2(DIFT2T0) -> rd_34/1
  signalquality/1(amoundofsyncs) -> rd_35/1
  CLKCNTER_ACT/1(CNT) -> OUTPUTCONTROLCONTINIOUS/1(CLKCNT), Compare To Constant3/1(u)
  OUTPUTCONTROLCONTINIOUS/1(CLKOFF) -> SetZeroBool/2(setzero), ManualSerialize/5(clkoff), Subsystem2/4(reset)
  OUTPUTCONTROLCONTINIOUS/2(DATAINV) -> Logical Operator4/1, Logical Operator14/1
  SetZeroBool/1(valueout) -> CLKCNTER_ACT/2(CLK2CNT), Delay4/1
  OUTPUTCONTROLCONTINIOUS/3(RESETCNT) -> CLKCNTER_NOSTOP/3(ResetCNT), CLKCNTER_ACT/3(ResetCNT)
  CLKCNTER_NOSTOP/1(CNT) -> OUTPUTCONTROLCONTINIOUS/5(CLKCNTNOSTOP)
  DATAFLOWCHGER/1(Output) -> OUTPUTCONTROLCONTINIOUS/2(CLKS2DATAFLOWCHG)
  Subsystem6/1(Out1) -> OUTPUTCONTROLCONTINIOUS/3(CLK2ENDOFTRANSMISSION)
  RECOVERYTIMESELECTOR/1(Out1) -> OUTPUTCONTROLCONTINIOUS/6(RECOVERYTIME)
  Dual Port RAM System/2 -> 8BIT_SPLITTER/1(DATAIN)
  FKT1DATAFLOW/1 -> RAM_SELECTOR1/4
  FKT2RECOVERYTIME/1 -> RAM_SELECTOR1/5
  FKT4DATACLKSYNC/1 -> RAM_SELECTOR1/6
  FKT5TELEGRAMLEN/1 -> RAM_SELECTOR1/7
  FKT6SYNCRESPONSE/1 -> RAM_SELECTOR1/8
  FKT7EXTRASHIFT/1 -> RAM_SELECTOR1/9
  TmpGroundAtRAM_SELECTOR1Inport10/1 -> RAM_SELECTOR1/10
  RAM_SELECTOR/1 -> Dual Port RAM System/2, Dual Port RAM System/4
  Logical Operator/1 -> Dual Port RAM System/3
  RAM_SELECTOR1/1 -> Signal Specification/1
  Signal Specification/1 -> Dual Port RAM System/1
  concat/1 -> rd_1/1
  8BIT_SPLITTER/1(DATAOUT0) -> CONTROLWORDSTORED/2(DATA)
  Compare To Constant2/1(y) -> CONTROLWORDSTORED/1(CLK)
  Data Type Conversion9/1 -> concatenate1/6
  Data Type Conversion8/1 -> concatenate1/5
  Data Type Conversion7/1 -> concatenate1/4
  Data Type Conversion6/1 -> concatenate1/3
  Data Type Conversion5/1 -> concatenate1/2
  Data Type Conversion4/1 -> concatenate1/1
  concatenate1/1 -> t3/1
  t3/1 -> concat/6
  t3/2 -> concat/5
  t3/3 -> concat/4
  t3/4 -> concat/3
  t3/5 -> concat/2
  t3/6 -> concat/1
  CONTROLWORDSTORED/6(DATAOUT5) -> Data Type Conversion9/1
  Logical Operator6/1 -> Logical Operator8/3
  rd_29/1 -> SENSORERROR/1
  rd_31/1 -> DBGPOSRAW/1
  rd_4/1 -> Logical Operator8/1
  rd_0/1 -> ramselektor/1(In1)
  rd_5/1 -> Logical Operator8/2
  rd_33/1 -> DIFT0T1BUS/1
  rd_34/1 -> DIFT0T2BUS/1
  rd_17/1 -> SetZeroBool4/1(valin)
  rd_27/1 -> DBGREADPULSES/1
  rd_28/1 -> DBGWRITEOKPULSE/1
  rd_19/1 -> CRCEXTRACTED0/1
  rd_22/1 -> CRCEXTRACTED1/1
  rd_24/1 -> CRCEXTRACTED2/1
  rd_26/1 -> DBGACTIVENUMBER/1
  rd_16/1 -> clkwr/1
  rd_35/1 -> SYNCQUALITYBUS/1
  rd_21/1 -> CRCFFSTORED/1
  rd_6/1 -> OUTPUTCONTROLCONTINIOUS/4(OPENCOM)
  rd_1/1 -> RAM_SELECTOR1/3
  rd_7/1 -> Subsystem2/3(DATA)
  rd_12/1 -> statusword/1
  rd_11/1 -> multiportswitch1/2
  rd_10/1 -> multiportswitch1/1
  rd_32/1 -> DBGDATAIN/1
  Logical Operator22/1 -> SetZeroBool5/Trigger, SetZeroBool2/Trigger, INITIALOFF/2(CLK), rd_14/1
  rd_14/1 -> SetZeroBool4/Trigger, SetZeroBool3/Trigger
  Multiport Switch/1 -> rd_2/1
  rd_2/1 -> CLKCNTER_NOSTOP/2(CLK2CNT), Subsystem2/2(SLOWCLCK), SetZeroBool/1(valin), SetZeroBool/Trigger
  CLK50MHZ/1 -> 8BIT_SPLITTER/Trigger, ramselektor/Trigger, CONTROLWORDRAW/1(CLK), CLKDIV1/1(CLK1), Subsystem/1(CLK), CRC_Check/3(clk), ManualSerialize/1(CLK), timingprovider/2(clk), rd_3/1
  rd_3/1 -> SetZeroBool1/Trigger, Subsystem2/1(CLK), CLKCNTER_NOSTOP/1(CLK), CLKCNTER_ACT/1(CLK)
  Logical Operator27/1 -> rd_8/1
  rd_8/1 -> SetZeroBool2/2(setzero), SetZeroBool5/2(setzero), rd_13/1
  rd_13/1 -> SetZeroBool4/2(setzero), SetZeroBool3/2(setzero)
  RESPONSESLICER3X/4(payload1) -> DIFFBUILDER/2(DATAT1), rd_23/1
  rd_23/1 -> POS1BUS/1, POS1/1
  RESPONSESLICER3X/6(payload2) -> DIFFBUILDER/3(DATAT2), rd_25/1
  rd_25/1 -> POS2BUS/1, POS2/1
  RESPONSESLICER3X/2(payload) -> DIFFBUILDER/1(DATAT0), rd_20/1
  rd_20/1 -> DBGPOSSLICED/1, POS0BUS/1, POS0/1
  multiportswitch/1 -> ManualSerialize/2(SLOWCLCK), rd_9/1
  rd_9/1 -> DBGCLK/1, CLK_OUT/1
  SetZeroBool4/1(valueout) -> rd_18/1
  rd_18/1 -> DBGDATWRITE/1, datawr/1
  SetZeroBool3/1(valueout) -> rd_15/1
  rd_15/1 -> dataout/1, DBGDATAOUT/1
  ManualSerialize/4(dbg2) -> rd_30/1
  rd_30/1 -> RESPONSELENBUS/1, DBGTOTALBITSREAD/1

== system gm_UZ_EnDat/ENDAT23BITREVERSER1/16BITREVERSER ==
  in : Inport
  Bit Concat : hdlsllib/Logic and Bit Operations/Bit Concat  numInputs=4
  Bit Slice : hdlsllib/Logic and Bit Operations/Bit Slice  lidx=3  ridx=0
  Bit Slice1 : hdlsllib/Logic and Bit Operations/Bit Slice  lidx=7  ridx=4
  Bit Slice2 : hdlsllib/Logic and Bit Operations/Bit Slice  lidx=11  ridx=8
  Bit Slice3 : hdlsllib/Logic and Bit Operations/Bit Slice  lidx=15  ridx=12
  out : Outport
  wires:
  Bit Concat/1 -> out/1
  Bit Slice3/1 -> Bit Concat/4
  Bit Slice2/1 -> Bit Concat/3
  Bit Slice/1 -> Bit Concat/1
  Bit Slice1/1 -> Bit Concat/2
  in/1 -> Bit Slice1/1, Bit Slice2/1, Bit Slice3/1, Bit Slice/1

== system gm_UZ_EnDat/ENDAT23BITREVERSER1/16BITREVERSER1 ==
  in : Inport
  Bit Concat : hdlsllib/Logic and Bit Operations/Bit Concat  numInputs=4
  Bit Slice : hdlsllib/Logic and Bit Operations/Bit Slice  lidx=3  ridx=0
  Bit Slice1 : hdlsllib/Logic and Bit Operations/Bit Slice  lidx=7  ridx=4
  Bit Slice2 : hdlsllib/Logic and Bit Operations/Bit Slice  lidx=11  ridx=8
  Bit Slice3 : hdlsllib/Logic and Bit Operations/Bit Slice  lidx=15  ridx=12
  out : Outport
  wires:
  Bit Concat/1 -> out/1
  Bit Slice3/1 -> Bit Concat/4
  Bit Slice2/1 -> Bit Concat/3
  Bit Slice/1 -> Bit Concat/1
  Bit Slice1/1 -> Bit Concat/2
  in/1 -> Bit Slice1/1, Bit Slice2/1, Bit Slice3/1, Bit Slice/1

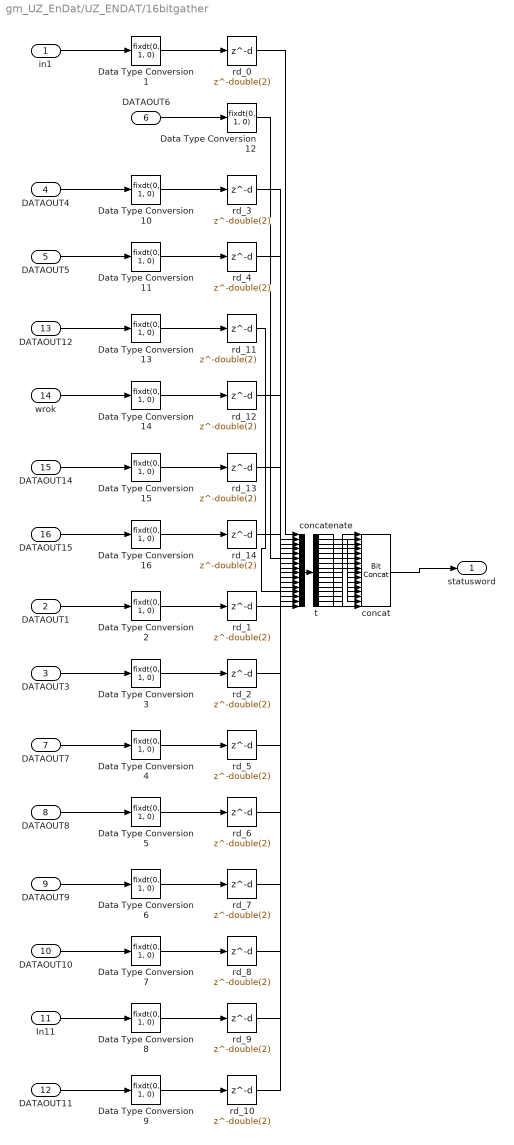
== system gm_UZ_EnDat/UZ_ENDAT/16bitgather ==
  in1 : Inport  OutDataTypeStr=boolean  PortDimensions=1  SampleTime=1e-08
  DATAOUT1 : Inport  Port=2  OutDataTypeStr=boolean  PortDimensions=1  SampleTime=1e-08
  DATAOUT3 : Inport  Port=3  OutDataTypeStr=boolean  PortDimensions=1  SampleTime=1e-08
  DATAOUT4 : Inport  Port=4  OutDataTypeStr=boolean  PortDimensions=1  SampleTime=1e-08
  DATAOUT5 : Inport  Port=5  OutDataTypeStr=boolean  PortDimensions=1  SampleTime=1e-08
  DATAOUT6 : Inport  Port=6  OutDataTypeStr=boolean  PortDimensions=1  SampleTime=1e-08
  DATAOUT7 : Inport  Port=7  OutDataTypeStr=boolean  PortDimensions=1  SampleTime=1e-08
  DATAOUT8 : Inport  Port=8  OutDataTypeStr=boolean  PortDimensions=1  SampleTime=1e-08
  DATAOUT9 : Inport  Port=9  OutDataTypeStr=boolean  PortDimensions=1  SampleTime=1e-08
  DATAOUT10 : Inport  Port=10  OutDataTypeStr=boolean  PortDimensions=1  SampleTime=1e-08
  In11 : Inport  Port=11  OutDataTypeStr=boolean  PortDimensions=1  SampleTime=1e-08
  DATAOUT11 : Inport  Port=12  OutDataTypeStr=boolean  PortDimensions=1  SampleTime=1e-08
  DATAOUT12 : Inport  Port=13  OutDataTypeStr=boolean  PortDimensions=1  SampleTime=1e-08
  wrok : Inport  Port=14  OutDataTypeStr=boolean  PortDimensions=1  SampleTime=1e-08
  DATAOUT14 : Inport  Port=15  OutDataTypeStr=boolean  PortDimensions=1  SampleTime=1e-08
  DATAOUT15 : Inport  Port=16  OutDataTypeStr=boolean  PortDimensions=1  SampleTime=1e-08
  Data Type Conversion{1..16} (16 alike) : DataTypeConversion  OutDataTypeStr=fixdt(0, 1, 0)  SampleTime=1e-08  SaturateOnIntegerOverflow=off  RndMeth=Floor
  concat : hdlsllib/Logic and Bit Operations/Bit Concat  numInputs=16
  concatenate : Concatenate  NumInputs=16
  rd_{0..14} (15 alike) : Delay  DelayLength=double(2)  InitialCondition=0  SampleTime=1e-08
  t : Demux  Outputs=16
  statusword : Outport  SampleTime=1e-08
  wires:
  in1/1 -> Data Type Conversion1/1
  DATAOUT1/1 -> Data Type Conversion2/1
  DATAOUT3/1 -> Data Type Conversion3/1
  DATAOUT4/1 -> Data Type Conversion10/1
  DATAOUT5/1 -> Data Type Conversion11/1
  DATAOUT6/1 -> Data Type Conversion12/1
  DATAOUT7/1 -> Data Type Conversion4/1
  DATAOUT8/1 -> Data Type Conversion5/1
  DATAOUT9/1 -> Data Type Conversion6/1
  DATAOUT10/1 -> Data Type Conversion7/1
  In11/1 -> Data Type Conversion8/1
  DATAOUT11/1 -> Data Type Conversion9/1
  DATAOUT12/1 -> Data Type Conversion13/1
  wrok/1 -> Data Type Conversion14/1
  DATAOUT14/1 -> Data Type Conversion15/1
  DATAOUT15/1 -> Data Type Conversion16/1
  concat/1 -> statusword/1
  Data Type Conversion12/1 -> concatenate/6
  concatenate/1 -> t/1
  t/1 -> concat/16
  t/2 -> concat/15
  t/3 -> concat/14
  t/4 -> concat/13
  t/5 -> concat/12
  t/6 -> concat/11
  t/7 -> concat/10
  t/8 -> concat/9
  t/9 -> concat/8
  t/10 -> concat/7
  t/11 -> concat/6
  t/12 -> concat/5
  t/13 -> concat/4
  t/14 -> concat/3
  t/15 -> concat/2
  t/16 -> concat/1
  Data Type Conversion1/1 -> rd_0/1
  Data Type Conversion2/1 -> rd_1/1
  Data Type Conversion3/1 -> rd_2/1
  Data Type Conversion10/1 -> rd_3/1
  Data Type Conversion11/1 -> rd_4/1
  Data Type Conversion4/1 -> rd_5/1
  Data Type Conversion5/1 -> rd_6/1
  Data Type Conversion6/1 -> rd_7/1
  Data Type Conversion7/1 -> rd_8/1
  Data Type Conversion8/1 -> rd_9/1
  Data Type Conversion9/1 -> rd_10/1
  Data Type Conversion13/1 -> rd_11/1
  Data Type Conversion14/1 -> rd_12/1
  Data Type Conversion15/1 -> rd_13/1
  Data Type Conversion16/1 -> rd_14/1
  rd_0/1 -> concatenate/1
  rd_3/1 -> concatenate/4
  rd_4/1 -> concatenate/5
  rd_11/1 -> concatenate/13
  rd_12/1 -> concatenate/14
  rd_13/1 -> concatenate/15
  rd_14/1 -> concatenate/16
  rd_1/1 -> concatenate/2
  rd_2/1 -> concatenate/3
  rd_5/1 -> concatenate/7
  rd_6/1 -> concatenate/8
  rd_7/1 -> concatenate/9
  rd_8/1 -> concatenate/10
  rd_9/1 -> concatenate/11
  rd_10/1 -> concatenate/12

== system gm_UZ_EnDat/UZ_ENDAT/3timestorage ==
  DATA : Inport  OutDataTypeStr=fixdt(0, 64, 0)  PortDimensions=1  SampleTime=1e-08
  wrok : Inport  Port=2  OutMin=0  OutMax=1  OutDataTypeStr=boolean  PortDimensions=1  SampleTime=1e-08
  Compare To Constant : Subsystem  mask(Compare To Constant){relop===, const=double(0), OutDataTypeStr=boolean, ZeroCross=on}
      mask prompts: relop "Simulink:masks:Operator_MP"; const "Simulink:masks:ConstantValue_MP"; OutDataTypeStr "Simulink:masks:OutputDataType_MP"; ZeroCross "Simulink:masks:EnableZerocrossingDetection_MP"
      mask help: Simulink:masks:CompareToConstant_MD
      mask TypeOptions relop: == | ~= | < | <= | >= | >
      mask TypeOptions OutDataTypeStr: Simulink:masks:uint8 | Simulink:masks:boolean
      mask Callback ZeroCross: sl('zeroCrossEnable', gcbh);
      mask Display: disp(str)
  Compare To Constant1 : Subsystem  mask(Compare To Constant){relop===, const=double(1), OutDataTypeStr=boolean, ZeroCross=on}
      mask prompts: relop "Simulink:masks:Operator_MP"; const "Simulink:masks:ConstantValue_MP"; OutDataTypeStr "Simulink:masks:OutputDataType_MP"; ZeroCross "Simulink:masks:EnableZerocrossingDetection_MP"
      mask help: Simulink:masks:CompareToConstant_MD
      mask init:
      | OutDataTypeStr = 'boolean';
      | ZeroCross = 'on';
      | blkName = 'UZ_EnDat/UZ_ENDAT/3timestorage/Compare\nTo Constant1';
      | const = double(1);
      | const_str = '1';
      | const_val = double(1);
      | relop = '==';
      | setValue = 'boolean';
      | str = '== 1';
      mask TypeOptions relop: == | ~= | < | <= | >= | >
      mask TypeOptions OutDataTypeStr: Simulink:masks:uint8 | Simulink:masks:boolean
      mask Callback ZeroCross: sl('zeroCrossEnable', gcbh);
      mask Display: disp(str)
  Compare To Constant2 : Subsystem  mask(Compare To Constant){relop===, const=double(2), OutDataTypeStr=boolean, ZeroCross=on}
      mask prompts: relop "Simulink:masks:Operator_MP"; const "Simulink:masks:ConstantValue_MP"; OutDataTypeStr "Simulink:masks:OutputDataType_MP"; ZeroCross "Simulink:masks:EnableZerocrossingDetection_MP"
      mask help: Simulink:masks:CompareToConstant_MD
      mask init:
      | OutDataTypeStr = 'boolean';
      | ZeroCross = 'on';
      | blkName = 'UZ_EnDat/UZ_ENDAT/3timestorage/Compare\nTo Constant2';
      | const = double(2);
      | const_str = '2';
      | const_val = double(2);
      | relop = '==';
      | setValue = 'boolean';
      | str = '== 2';
      mask TypeOptions relop: == | ~= | < | <= | >= | >
      mask TypeOptions OutDataTypeStr: Simulink:masks:uint8 | Simulink:masks:boolean
      mask Callback ZeroCross: sl('zeroCrossEnable', gcbh);
      mask Display: disp(str)
  Detect Increase2 : Subsystem  mask(Detect Increase){vinit=double(0), InputProcessing=Elements as channels (sample based), OutDataTypeStr=boolean}
      mask prompts: vinit "Simulink:masks:InitialCondition_MP"; InputProcessing "Simulink:masks:InputProcessing_MP"; OutDataTypeStr "Simulink:masks:OutputDataType_MP"
      mask help: Simulink:masks:DetectIncrease_MD
      mask TypeOptions InputProcessing: Simulink:masks:ColumnsAsChannelsFrameBased | Simulink:masks:ElementsAsChannelsSampleBased
      mask TypeOptions OutDataTypeStr: Simulink:masks:uint8 | Simulink:masks:boolean
      mask Display: fprintf('U > U/z')
  Detect Increase3 : Subsystem  mask(Detect Increase){vinit=double(0), InputProcessing=Elements as channels (sample based), OutDataTypeStr=boolean}
      mask prompts: vinit "Simulink:masks:InitialCondition_MP"; InputProcessing "Simulink:masks:InputProcessing_MP"; OutDataTypeStr "Simulink:masks:OutputDataType_MP"
      mask help: Simulink:masks:DetectIncrease_MD
      mask TypeOptions InputProcessing: Simulink:masks:ColumnsAsChannelsFrameBased | Simulink:masks:ElementsAsChannelsSampleBased
      mask TypeOptions OutDataTypeStr: Simulink:masks:uint8 | Simulink:masks:boolean
      mask Display: fprintf('U > U/z')
  Detect Increase4 : Subsystem  mask(Detect Increase){vinit=double(0), InputProcessing=Elements as channels (sample based), OutDataTypeStr=boolean}
      mask prompts: vinit "Simulink:masks:InitialCondition_MP"; InputProcessing "Simulink:masks:InputProcessing_MP"; OutDataTypeStr "Simulink:masks:OutputDataType_MP"
      mask help: Simulink:masks:DetectIncrease_MD
      mask TypeOptions InputProcessing: Simulink:masks:ColumnsAsChannelsFrameBased | Simulink:masks:ElementsAsChannelsSampleBased
      mask TypeOptions OutDataTypeStr: Simulink:masks:uint8 | Simulink:masks:boolean
      mask Display: fprintf('U > U/z')
  Multiport Switch : MultiPortSwitch  DataPortOrder=Zero-based contiguous  DiagnosticForDefault=None  zeroidx=on  OutDataTypeStr=fixdt(0, 64, 0)  RndMeth=Simplest  SampleTime=1e-08  SaturateOnIntegerOverflow=off  InputSameDT=off
  Multiport Switch1 : MultiPortSwitch  DataPortOrder=Zero-based contiguous  DiagnosticForDefault=None  zeroidx=on  OutDataTypeStr=fixdt(0, 64, 0)  RndMeth=Simplest  SampleTime=1e-08  SaturateOnIntegerOverflow=off  InputSameDT=off
  Multiport Switch2 : MultiPortSwitch  DataPortOrder=Zero-based contiguous  DiagnosticForDefault=None  zeroidx=on  OutDataTypeStr=fixdt(0, 64, 0)  RndMeth=Simplest  SampleTime=1e-08  SaturateOnIntegerOverflow=off  InputSameDT=off
  Storage1 : Subsystem
  Storage2 : Subsystem
  Storage20 : Subsystem
  Triggered Subsystem : Subsystem
  t0 : Outport  SampleTime=1e-08
  t-1 : Outport  Port=2  SampleTime=1e-08
  t-2 : Outport  Port=3  SampleTime=1e-08
  wires:
  DATA/1 -> Storage2/1(Data), Storage1/1(Data), Storage20/1(Data)
  wrok/1 -> Triggered Subsystem/Trigger
  Compare To Constant/1(y) -> Detect Increase4/1(U)
  Compare To Constant1/1(y) -> Detect Increase3/1(U)
  Compare To Constant2/1(y) -> Detect Increase2/1(U)
  Detect Increase2/1(Y) -> Storage2/2(Write)
  Detect Increase3/1(Y) -> Storage1/2(Write)
  Detect Increase4/1(Y) -> Storage20/2(Write)
  Multiport Switch/1 -> t0/1
  Multiport Switch1/1 -> t-1/1
  Multiport Switch2/1 -> t-2/1
  Storage1/1(out) -> Multiport Switch2/2, Multiport Switch1/4, Multiport Switch/3
  Storage2/1(out) -> Multiport Switch2/3, Multiport Switch1/2, Multiport Switch/4
  Storage20/1(out) -> Multiport Switch2/4, Multiport Switch1/3, Multiport Switch/2
  Triggered Subsystem/1(Out1) -> Multiport Switch2/1, Multiport Switch1/1, Multiport Switch/1, Compare To Constant/1(u), Compare To Constant1/1(u), Compare To Constant2/1(u)
